simulink model "mot_sim2"  (Simulink 4.00)
settings: Solver=ode45  SolverMode=SingleTasking  StartTime=0.0  StopTime=3  MaxStep=0.1  RelTol=1e-3  AbsTol=1e-3
values from neighbouring files (symbols this model uses):
  b = 0.1    [MOTOR.M]
  J = 0.01    [MOTOR.M]
  K = 0.01    [MOTOR.M]
  L = 0.5    [MOTOR.M]
  R = 1    [MOTOR.M]
settings Model: LastModifiedBy=R.Babuska  SaveTime=off  SaveOutput=off  LimitDataPoints=off  RTWTemplateMakefile=grt_vc.tmf

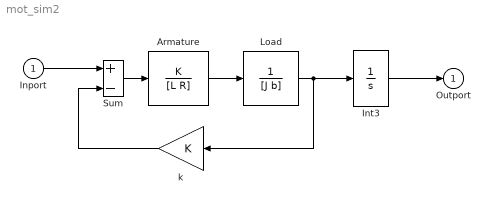
== system mot_sim2 ==
  Inport : Inport  Port=1  LatchInput=off
  " k " : Gain  Orientation=left  Gain=K  Multiplication=Element-wise(K.*u)  SaturateOnIntegerOverflow=on
  Armature : TransferFcn  Numerator=K  Denominator=[L R]  AbsoluteTolerance=auto  Realization=auto
  Int3 : Integrator  ExternalReset=none  InitialConditionSource=internal  InitialCondition=0  LimitOutput=off  UpperSaturationLimit=inf  LowerSaturationLimit=-inf  ShowSaturationPort=off  ShowStatePort=off  AbsoluteTolerance=auto
  Load : TransferFcn  Numerator=1  Denominator=[J b]  AbsoluteTolerance=auto  Realization=auto
  Sum : Sum  Inputs=+-  SaturateOnIntegerOverflow=on
  Outport : Outport  Port=1  InitialOutput=0
  wires:
  Int3/1 -> Outport/1
  Inport/1 -> Sum/1
  " k "/1 -> Sum/2
  Load/1 -> " k "/1, Int3/1
  Armature/1 -> Load/1
  Sum/1 -> Armature/1
